simulink model "x2"  (R2019b)
settings: Solver=VariableStepAuto  StartTime=0.0  StopTime=10.0  RelTol=1e-3
undefined symbols (not defined in the file): ini_x2, ini_x2_d, r2
settings Model: Creator=mic-ciciolla  LastModifiedBy=mic-ciciolla

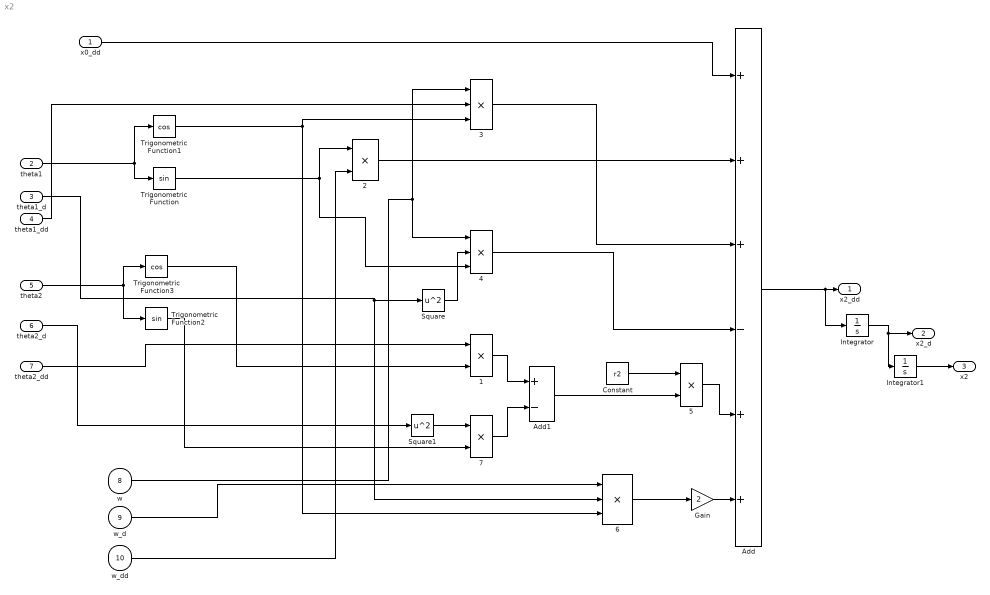
== system x2 ==
  x0_dd : Inport
  theta1 : Inport  Port=2
  theta1_d : Inport  Port=3
  theta1_dd : Inport  Port=4
  theta2 : Inport  Port=5
  theta2_d : Inport  Port=6
  "theta2_dd " : Inport  Port=7
  w : Inport  Port=8
  w_d : Inport  Port=9
  w_dd : Inport  Port=10
  {1..2,5,7} (4 alike) : Product
  3 : Product  Inputs=3
  4 : Product  Inputs=3
  6 : Product  Inputs=3
  Add : Sum  Inputs=+++-++
  Add1 : Sum  Inputs=+-
  Constant : Constant  Value=r2
  Gain : Gain  Gain=2
  Integrator : Integrator  InitialCondition=ini_x2_d
  Integrator1 : Integrator  InitialCondition=ini_x2
  Square : Math  Operator=square  SignedPower=off  SaturateOnIntegerOverflow=on
  Square1 : Math  Operator=square  SignedPower=off  SaturateOnIntegerOverflow=on
  Trigonometric Function : Trigonometry
  Trigonometric Function1 : Trigonometry  Operator=cos
  Trigonometric Function2 : Trigonometry
  Trigonometric Function3 : Trigonometry  Operator=cos
  x2_dd : Outport
  x2_d : Outport  Port=2
  x2 : Outport  Port=3
  wires:
  Add/1 -> Integrator/1, x2_dd/1
  Integrator/1 -> Integrator1/1, x2_d/1
  Integrator1/1 -> x2/1
  x0_dd/1 -> Add/1
  theta1/1 -> Trigonometric Function1/1, Trigonometric Function/1
  w_dd/1 -> 2/2
  Trigonometric Function/1 -> 4/3, 2/1
  theta2/1 -> Trigonometric Function3/1, Trigonometric Function2/1
  2/1 -> Add/2
  w/1 -> 3/1, 4/1
  theta1_dd/1 -> 3/2
  Trigonometric Function1/1 -> 6/3, 3/3
  3/1 -> Add/3
  4/1 -> Add/4
  theta1_d/1 -> 6/2, Square/1
  Square/1 -> 4/2
  Gain/1 -> Add/6
  6/1 -> Gain/1
  w_d/1 -> 6/1
  Constant/1 -> 5/1
  5/1 -> Add/5
  Add1/1 -> 5/2
  1/1 -> Add1/1
  7/1 -> Add1/2
  "theta2_dd "/1 -> 1/1
  Trigonometric Function3/1 -> 1/2
  theta2_d/1 -> Square1/1
  Square1/1 -> 7/1
  Trigonometric Function2/1 -> 7/2
